simulink model "halfmodel_improved"  (R2018b)
settings: Solver=VariableStepAuto  StartTime=0.0  StopTime=10  RelTol=1e-3
values from neighbouring files (symbols this model uses):
  a = 1.25    [initModel.m]
  b = 1.4    [initModel.m]
  bodySettle = frontBodySettle-((frontBodySettle-rearBodySettle)*(a/(a+b)))    (= -0.141993301633)    [initModel.m]
  csCompress = 600    [initModel.m]
  csExtend = 1200    [initModel.m]
  frontHoldForce = mb*g*b/(a+b)    (= 2591.32075472)    [initModel.m]
  frontWheelSettle = -(frontHoldForce+(m2*g))/kT    (= -0.0199108625337)    [initModel.m]
  g = 9.81    [initModel.m]
  I = 600    [initModel.m]
  ks = 2e4    (= 20000)    [initModel.m]
  ksHard = 20*ks    (= 400000)    [initModel.m]
  kT = 14e4    (= 140000)    [initModel.m]
  kTHard = 1e10    (= 10000000000)    [initModel.m]
  m2 = 20    [initModel.m]
  mb = 500    [initModel.m]
  pitchSettle = asin((frontBodySettle-rearBodySettle)/(a+b))    [initModel.m]
  rearHoldForce = mb*g*a/(a+b)    (= 2313.67924528)    [initModel.m]
  rearWheelSettle = -(rearHoldForce+(m2*g))/kT    (= -0.0179277088949)    [initModel.m]
  stepValue = -0.2    [initModel.m]
  tyreLimit = 0.15    [initModel.m]
  v_speed = 10    [initModel.m]
  x0 = 0.2    [initModel.m]
undefined symbols (not defined in the file or in its folder): initModel
libraries: simulink x1, dspsrcs4 x1
settings Model: SnapshotBufferSize=100  Creator=Jamie  LastModifiedBy=Jamie

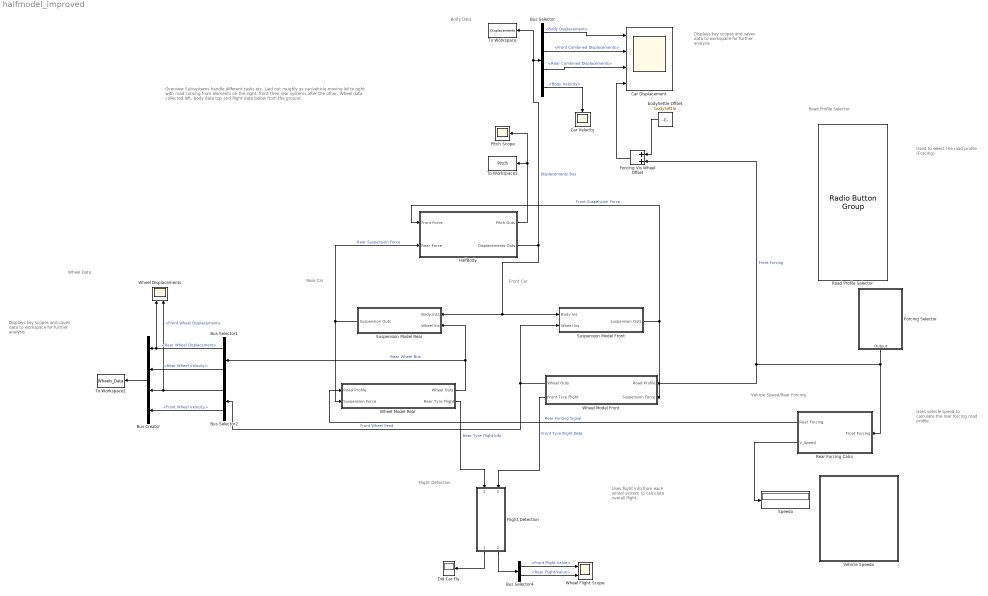
== system halfmodel_improved ==
  note: Used to select the road profile (Forcing)
  note: Vehicle Speed/Rear Forcing
  note: Flight Detection
  note: Road Profile Selector
  note: Wheel Data
  note: Front Car
  note: Rear Car
  note: Body Data
  note: Uses vehicle speed to calculate the rear forcing road profile
  note: Uses flight info from each wheel system to calculate overall flight.
  note: Displays key scopes and saves data to workspace for further analysis
  note: Displays key scopes and saves data to workspace for further analysis
  note: Overview
      | Subsystems handle different tasks etc. Laid out roughly as car/vehicle moving lef to right with road coming from elements on the right, front then rear systems after the other. Wheel data collected left, body data top and flight data below from the ground.
  Bus Creator : BusCreator  Inputs=4
  Bus Selector : BusSelector  OutputSignals=Body Displacement,Front Combined Displacements,Rear Combined Displacements,Body Velocity
  Bus Selector1 : BusSelector  OutputSignals=Rear Wheel Displacement,Rear Wheel Velocity
  Bus Selector2 : BusSelector  OutputSignals=Front Wheel Displacement,Front Wheel Velocity
  Bus Selector4 : BusSelector  OutputSignals=Front Flight Value,Rear Flight Value
  Car Displacement : Scope  NumInputPorts=4
  Car Velocity : Scope
  Did Car Fly : Display
  Flight Detection : Subsystem
  Forcing Selector : Subsystem
  Forcing Vis Wheel Offset : Sum
  HalfBody : Subsystem
  Pitch Scope : Scope
  Rear Forcing Calcs : Subsystem
  Road Profile Selector : RadioButtonGroup  LoadFcn=initModel;  WebBlockId=387  SelectedLabel=Random  ButtonGroupName=Road Input
      settings: Values={{'Step', 'Sin', 'Zero', 'Pulses', 'Humpback', 'Random'}, [1 2 3 4 5 6]}
  Speedo : Display
  Suspension Model Front : Subsystem
  Suspension Model Rear : Subsystem
  To Workspace : ToWorkspace  VariableName=Displacements  SaveFormat=Timeseries  SampleTime=-1
  To Workspace1 : ToWorkspace  VariableName=Wheels_Data  SaveFormat=Timeseries  SampleTime=-1
  To Workspace3 : ToWorkspace  VariableName=Pitch  SaveFormat=Timeseries  SampleTime=-1
  Vehicle Speedo : Subsystem  Description=Replaced Block  mask(Replaced Block){}
      mask help: This block has been replaced with an empty subsystem because it used functionality that is unavailable in Simulink R2017b.
      mask Display: fprintf('Unavailable in 2017b. \nSee report for info\nand screenshot')
  Wheel Displacements : Scope  NumInputPorts=2
  Wheel Flight Scope : Scope  NumInputPorts=2
  Wheel Model Front : Subsystem
  Wheel Model Rear : Subsystem
  bodySettle Offset : Constant  Value=bodySettle
  wires:
  HalfBody/2(Displacements Outs) -> To Workspace/1, Bus Selector/1, Suspension Model Front/1(Body Ins), Suspension Model Rear/1(Body Ins1)  "Displacements Bus"
  Suspension Model Rear/1(Suspension Outs) -> HalfBody/2(Rear Force), Wheel Model Rear/2(Suspension Force)  "Rear Suspension Force"
  Wheel Model Rear/1(Wheel Outs) -> Suspension Model Rear/2(Wheel Ins), Bus Selector1/1  "Rear Wheel Bus"
  Wheel Model Front/1(Wheel Outs) -> Bus Selector2/1, Suspension Model Front/2(Wheel Ins)  "Front Wheel Feed"
  Suspension Model Front/1(Suspension Outs) -> Wheel Model Front/2(Suspension Force), HalfBody/1(Front Force)  "Front Suspension Force"
  Forcing Selector/1(Output) -> Rear Forcing Calcs/1(Front Forcing), Forcing Vis Wheel Offset/2, Wheel Model Front/1(Road Profile)  "Front Forcing"
  Rear Forcing Calcs/1(Rear Forcing) -> Wheel Model Rear/1(Road Profile)  "Rear Forcing Signal"
  Bus Selector/4 -> Car Velocity/1  "<Body Velocity>"
  Bus Selector/1 -> Car Displacement/1  "<Body Displacement>"
  HalfBody/1(Pitch Outs) -> Pitch Scope/1, To Workspace3/1
  Bus Selector1/1 -> Wheel Displacements/1, Bus Creator/1  "<Rear Wheel Displacement>"
  Bus Selector1/2 -> Bus Creator/2  "<Rear Wheel Velocity>"
  Bus Creator/1 -> To Workspace1/1
  Bus Selector2/1 -> Wheel Displacements/2, Bus Creator/3  "<Front Wheel Displacement>"
  Bus Selector2/2 -> Bus Creator/4  "<Front Wheel Velocity>"
  Forcing Vis Wheel Offset/1 -> Car Displacement/4
  bodySettle Offset/1 -> Forcing Vis Wheel Offset/1
  Wheel Model Front/2(Front Tyre Flight) -> Flight Detection/2(Wheel 2 Data)  "Front Tyre Flight Data"
  Wheel Model Rear/2(Rear Tyre Flight) -> Flight Detection/1(Wheel 1 Data)  "Rear Tyre Flight Info"
  Flight Detection/1(Car Flight) -> Did Car Fly/1
  Flight Detection/2(Wheel Flights) -> Bus Selector4/1
  Bus Selector4/1 -> Wheel Flight Scope/1  "<Front Flight Value>"
  Bus Selector4/2 -> Wheel Flight Scope/2  "<Rear Flight Value>"
  Rear Forcing Calcs/2(V_Speed) -> Speedo/1
  Bus Selector/2 -> Car Displacement/2  "<Front Combined Displacements>"
  Bus Selector/3 -> Car Displacement/3  "<Rear Combined Displacements>"

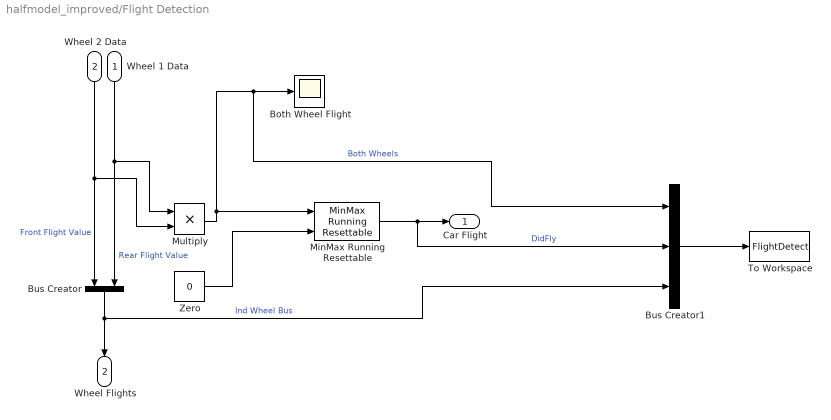
== system halfmodel_improved/Flight Detection ==
  Wheel 1 Data : Inport
  Wheel 2 Data : Inport  Port=2
  Both Wheel Flight : Scope
  Bus Creator : BusCreator  Inputs=2
  Bus Creator1 : BusCreator  Inputs=3
  MinMax Running Resettable : simulink/Math Operations/MinMax Running Resettable  Function=max  vinit=0
  Multiply : Product
  To Workspace : ToWorkspace  VariableName=FlightDetect  SaveFormat=Timeseries  SampleTime=-1
  Zero : Constant  Value=0  OutDataTypeStr=Inherit: Inherit via back propagation
  Car Flight : Outport
  Wheel Flights : Outport  Port=2
  wires:
  Wheel 1 Data/1 -> Multiply/1, Bus Creator/2  "Rear Flight Value"
  Wheel 2 Data/1 -> Multiply/2, Bus Creator/1  "Front Flight Value"
  MinMax Running Resettable/1 -> Bus Creator1/2, Car Flight/1  "DidFly"
  Multiply/1 -> Bus Creator1/1, Both Wheel Flight/1, MinMax Running Resettable/1  "Both Wheels"
  Zero/1 -> MinMax Running Resettable/2
  Bus Creator/1 -> Bus Creator1/3, Wheel Flights/1  "Ind Wheel Bus"
  Bus Creator1/1 -> To Workspace/1

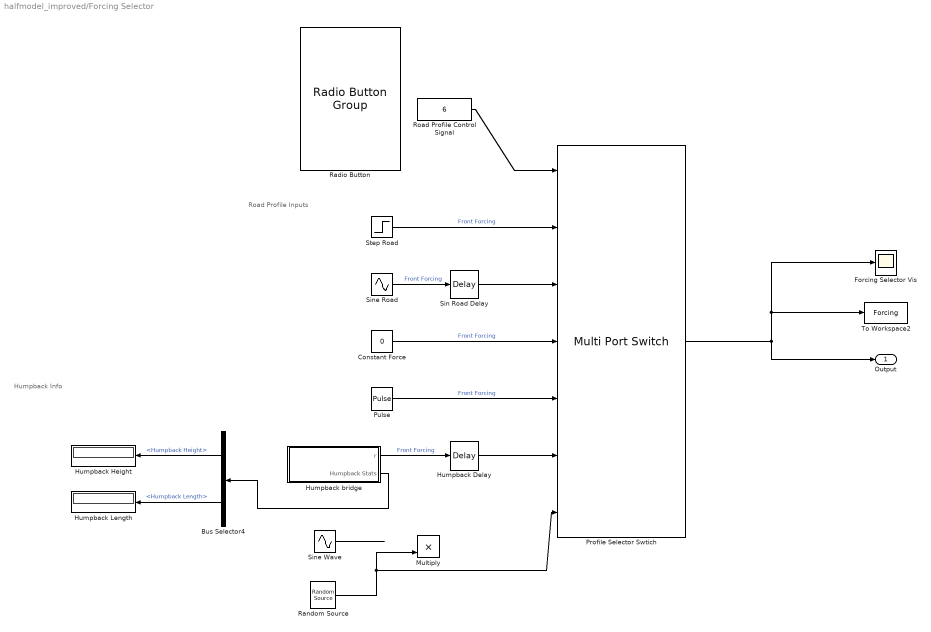
== system halfmodel_improved/Forcing Selector ==
  note: Humpback Info
  note: Road Profile Inputs
  Bus Selector4 : BusSelector  OutputSignals=Humpback Height,Humpback Length
  Constant Force : Constant  Value=0
  Forcing Selector Vis : Scope
  Humpback Delay : TransportDelay  BufferSize=4096
  Humpback bridge : Subsystem  mask{h=2, L=20, v=v_speed, startTime=0}
      mask prompts: h "humpback height (m)"; L "humpback length (m)"; v "vehicle speed (m/s)"; startTime "Humpback Start Time Multiplier"
  Humpback Height : Display
  Humpback Length : Display
  Multiply : Product
  Profile Selector Swtich : MultiPortSwitch  Inputs=6
  Pulse : DiscretePulseGenerator  PulseType=Time based  Amplitude=0.15  PulseWidth=5  PhaseDelay=1
  Radio Button : RadioButtonGroup  WebBlockId=386  SelectedLabel=Random  ButtonGroupName=Road Input
      settings: Values={{'Step', 'Sin', 'Zero', 'Pulses', 'Humpback', 'Random'}, [1 2 3 4 5 6]}
  Random Source : dspsrcs4/Random Source  SrcType=Uniform  NormMethod=Ziggurat  CltLength=12  MinVal=-0.03  MaxVal=0.03  MeanVal=0  VarVal=0.002  RepMode=Not repeatable  rawSeed=1  IsInherit=off  SampMode=Discrete  SampTime=1/20  SampFrame=1  DataType=Double  OutComplex=Real  OutputFrames=off
  Road Profile Control Signal : Constant  Value=6
  "Sin Road Delay " : TransportDelay
  Sine Road : Sin  Amplitude=0.01  Frequency=2*pi*v_speed  SampleTime=0
  Sine Wave : Sin  Frequency=2  SampleTime=0
  Step Road : Step  Time=5  After=stepValue  SampleTime=0
  To Workspace2 : ToWorkspace  VariableName=Forcing  SaveFormat=Timeseries  SampleTime=-1
  Output : Outport
  wires:
  Bus Selector4/2 -> Humpback Length/1  "<Humpback Length>"
  Bus Selector4/1 -> Humpback Height/1  "<Humpback Height>"
  Humpback bridge/2(Humpback Stats) -> Bus Selector4/1
  Step Road/1 -> Profile Selector Swtich/2  "Front Forcing"
  Sine Road/1 -> "Sin Road Delay "/1  "Front Forcing"
  Constant Force/1 -> Profile Selector Swtich/4  "Front Forcing"
  Pulse/1 -> Profile Selector Swtich/5  "Front Forcing"
  Humpback bridge/1(r) -> Humpback Delay/1  "Front Forcing"
  Road Profile Control Signal/1 -> Profile Selector Swtich/1
  Profile Selector Swtich/1 -> To Workspace2/1, Forcing Selector Vis/1, Output/1
  Humpback Delay/1 -> Profile Selector Swtich/6
  "Sin Road Delay "/1 -> Profile Selector Swtich/3
  Sine Wave/1 -> ?
  Random Source/1 -> Multiply/2, Profile Selector Swtich/7

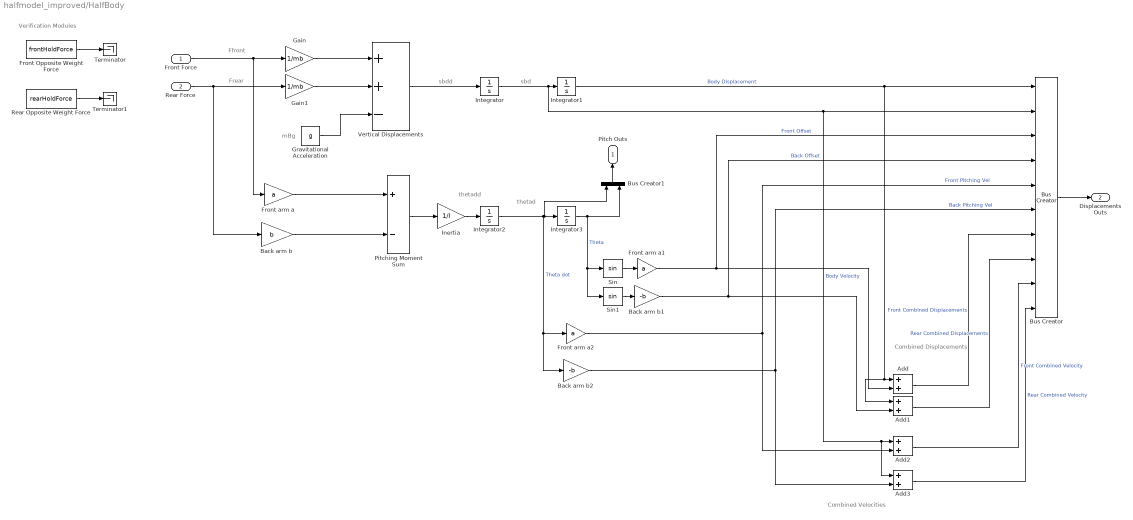
== system halfmodel_improved/HalfBody ==
  note: Combined Velocities
  note: Verification Modules
  note: thetadd
  note: Ffront
  note: Frear
  note: mBg
  note: sbdd
  note: sbd
  note: thetad
  note: Combined
      | Displacements
  Front Force : Inport
  Rear Force : Inport  Port=2
  Add{,1..3} (4 alike) : Sum
  Back arm b : Gain  Gain=b
  Back arm b1 : Gain  Gain=-b
  Back arm b2 : Gain  Gain=-b
  Bus Creator : BusCreator  Inputs=10
  Bus Creator1 : BusCreator  Inputs=2
  Front Opposite Weight Force : Constant  Value=frontHoldForce
  Front arm a : Gain  Gain=a
  Front arm a1 : Gain  Gain=a
  Front arm a2 : Gain  Gain=a
  Gain : Gain  Gain=1/mb
  Gain1 : Gain  Gain=1/mb
  Gravitational Acceleration : Constant  Value=g  mask{g=g}
      mask prompts: g "Gravitational Acceleration"
  Inertia : Gain  Gain=1/I
  Integrator : Integrator
  Integrator1 : Integrator  InitialCondition=bodySettle
  Integrator2 : Integrator
  Integrator3 : Integrator  InitialCondition=pitchSettle
  Pitching Moment Sum : Sum  Inputs=+-
  Rear Opposite Weight Force : Constant  Value=rearHoldForce
  Sin : Trigonometry
  Sin1 : Trigonometry
  Terminator : Terminator
  Terminator1 : Terminator
  Vertical Displacements : Sum  Inputs=++-
  Pitch Outs : Outport
  Displacements Outs : Outport  Port=2
  wires:
  Gravitational Acceleration/1 -> Vertical Displacements/3
  Gain/1 -> Vertical Displacements/1
  Gain1/1 -> Vertical Displacements/2
  Integrator1/1 -> Bus Creator/1, Add1/1, Add/1  "Body Displacement"
  Vertical Displacements/1 -> Integrator/1
  Integrator/1 -> Add2/1, Add3/1, Bus Creator/2, Integrator1/1  "Body Velocity"
  Back arm b/1 -> Pitching Moment Sum/2
  Front arm a/1 -> Pitching Moment Sum/1
  Pitching Moment Sum/1 -> Inertia/1
  Integrator2/1 -> Back arm b2/1, Front arm a2/1, Integrator3/1, Bus Creator1/1  "Theta dot"
  Inertia/1 -> Integrator2/1
  Bus Creator1/1 -> Pitch Outs/1
  Integrator3/1 -> Bus Creator1/2, Sin1/1, Sin/1  "Theta"
  Front arm a1/1 -> Add/2, Bus Creator/3  "Front Offset"
  Back arm b1/1 -> Add1/2, Bus Creator/4  "Back Offset"
  Bus Creator/1 -> Displacements Outs/1
  Front arm a2/1 -> Bus Creator/5, Add2/2  "Front Pitching Vel"
  Back arm b2/1 -> Bus Creator/6, Add3/2  "Back Pitching Vel"
  Sin/1 -> Front arm a1/1
  Sin1/1 -> Back arm b1/1
  Rear Force/1 -> Back arm b/1, Gain1/1
  Front Force/1 -> Gain/1, Front arm a/1
  Front Opposite Weight Force/1 -> Terminator/1
  Rear Opposite Weight Force/1 -> Terminator1/1
  Add/1 -> Bus Creator/7  "Front Combined Displacements"
  Add1/1 -> Bus Creator/8  "Rear Combined Displacements"
  Add2/1 -> Bus Creator/9  "Front Combined Velocity"
  Add3/1 -> Bus Creator/10  "Rear Combined Velocity"

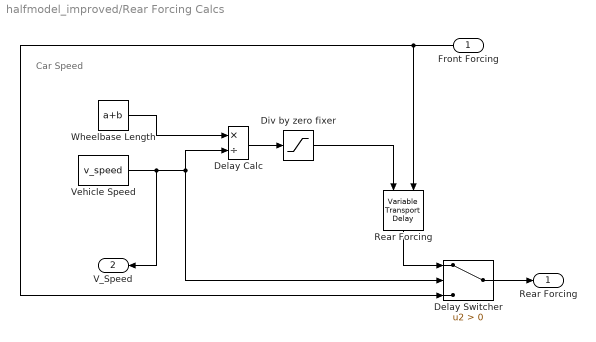
== system halfmodel_improved/Rear Forcing Calcs ==
  note: Car Speed
  Front Forcing : Inport
  Delay Calc : Product  Inputs=*/
  Delay Switcher : Switch  Criteria=u2 > Threshold
  Div by zero fixer : Saturate  UpperLimit=60  LowerLimit=0
  "Rear Forcing " : VariableTransportDelay  VariableDelayType=Variable transport delay  MaximumDelay=60  MaximumPoints=8192
  Vehicle Speed : Constant  Value=v_speed
  Wheelbase Length : Constant  Value=a+b
  Rear Forcing : Outport
  V_Speed : Outport  Port=2
  wires:
  Vehicle Speed/1 -> V_Speed/1, Delay Switcher/2, Delay Calc/2
  Delay Calc/1 -> Div by zero fixer/1
  Front Forcing/1 -> "Rear Forcing "/1, Delay Switcher/3
  Delay Switcher/1 -> Rear Forcing/1
  Wheelbase Length/1 -> Delay Calc/1
  "Rear Forcing "/1 -> Delay Switcher/1
  Div by zero fixer/1 -> "Rear Forcing "/2

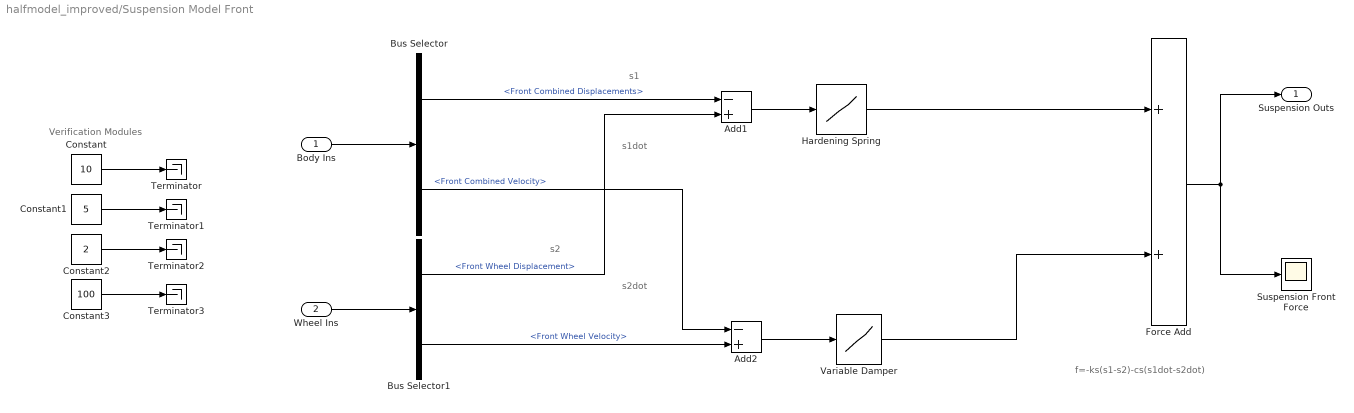
== system halfmodel_improved/Suspension Model Front ==
  note: Verification Modules
  note: s2dot
  note: s2
  note: f=-ks(s1-s2)-cs(s1dot-s2dot)
  note: s1dot
  note: s1
  Body Ins : Inport
  Wheel Ins : Inport  Port=2
  Add1 : Sum  Inputs=-+
  Add2 : Sum  Inputs=-+
  Bus Selector : BusSelector  OutputSignals=Front Combined Displacements,Front Combined Velocity
  Bus Selector1 : BusSelector  OutputSignals=Front Wheel Displacement,Front Wheel Velocity
  Constant : Constant  Value=10
  Constant1 : Constant  Value=5
  Constant2 : Constant  Value=2
  Constant3 : Constant  Value=100
  "Force Add " : Sum
  Hardening Spring : Lookup_n-D  NumberOfTableDimensions=1  BreakpointsForDimension1=[-2*x0,-1.5*x0,-x0,x0,1.5*x0,2*x0]  Table=[-1e10,-(ks+(ksHard/2))*x0,-ks*x0,ks*x0,(ks+(ksHard/2))*x0,1e10]  InternalRulePriority=Speed  RndMeth=Simplest  InputSameDT=on
  Suspension Front Force : Scope
  Terminator{,1..3} (4 alike) : Terminator
  Variable Damper : Lookup_n-D  NumberOfTableDimensions=1  BreakpointsForDimension1=[-1,0,1]  Table=[-csExtend,0,csCompress]  InternalRulePriority=Speed  RndMeth=Simplest  InputSameDT=on
  Suspension Outs : Outport
  wires:
  Body Ins/1 -> Bus Selector/1
  Wheel Ins/1 -> Bus Selector1/1
  Bus Selector1/2 -> Add2/2  "<Front Wheel Velocity>"
  Bus Selector1/1 -> Add1/2  "<Front Wheel Displacement>"
  "Force Add "/1 -> Suspension Front Force/1, Suspension Outs/1
  Bus Selector/1 -> Add1/1  "<Front Combined Displacements>"
  Bus Selector/2 -> Add2/1  "<Front Combined Velocity>"
  Constant/1 -> Terminator/1
  Constant1/1 -> Terminator1/1
  Constant2/1 -> Terminator2/1
  Constant3/1 -> Terminator3/1
  Hardening Spring/1 -> "Force Add "/1
  Add2/1 -> Variable Damper/1
  Variable Damper/1 -> "Force Add "/2
  Add1/1 -> Hardening Spring/1

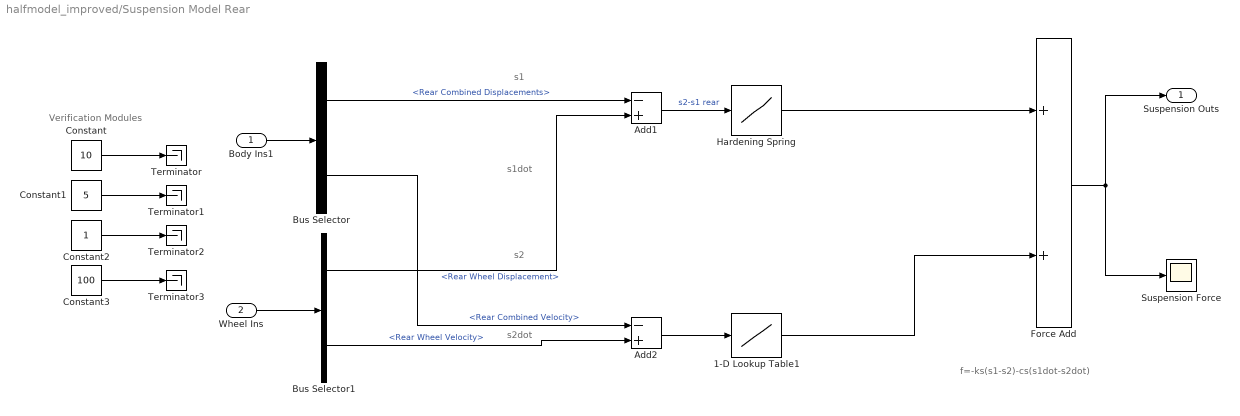
== system halfmodel_improved/Suspension Model Rear ==
  note: Verification Modules
  note: s2dot
  note: s2
  note: f=-ks(s1-s2)-cs(s1dot-s2dot)
  note: s1dot
  note: s1
  Body Ins1 : Inport
  Wheel Ins : Inport  Port=2
  1-D Lookup Table1 : Lookup_n-D  NumberOfTableDimensions=1  BreakpointsForDimension1=[-1,0,1]  Table=[-csExtend,0,csCompress]  InternalRulePriority=Speed  RndMeth=Simplest  InputSameDT=on
  Add1 : Sum  Inputs=-+
  Add2 : Sum  Inputs=-+
  Bus Selector : BusSelector  OutputSignals=Rear Combined Displacements,Rear Combined Velocity
  Bus Selector1 : BusSelector  OutputSignals=Rear Wheel Displacement,Rear Wheel Velocity
  Constant : Constant  Value=10
  Constant1 : Constant  Value=5
  Constant2 : Constant
  Constant3 : Constant  Value=100
  "Force Add " : Sum
  Hardening Spring : Lookup_n-D  NumberOfTableDimensions=1  BreakpointsForDimension1=[-2*x0,-1.5*x0,-x0,x0,1.5*x0,2*x0]  Table=[-1e10,-(ks+(ksHard/2))*x0,-ks*x0,ks*x0,(ks+(ksHard/2))*x0,1e10]  InternalRulePriority=Speed  RndMeth=Simplest  InputSameDT=on
  Suspension Force : Scope
  Terminator{,1..3} (4 alike) : Terminator
  Suspension Outs : Outport
  wires:
  Bus Selector1/2 -> Add2/2  "<Rear Wheel Velocity>"
  Bus Selector1/1 -> Add1/2  "<Rear Wheel Displacement>"
  "Force Add "/1 -> Suspension Force/1, Suspension Outs/1
  Body Ins1/1 -> Bus Selector/1
  Bus Selector/1 -> Add1/1  "<Rear Combined Displacements>"
  Wheel Ins/1 -> Bus Selector1/1
  Constant3/1 -> Terminator3/1
  Constant1/1 -> Terminator1/1
  Constant2/1 -> Terminator2/1
  Constant/1 -> Terminator/1
  1-D Lookup Table1/1 -> "Force Add "/2
  Hardening Spring/1 -> "Force Add "/1
  Add2/1 -> 1-D Lookup Table1/1
  Add1/1 -> Hardening Spring/1  "s2-s1 rear"
  Bus Selector/2 -> Add2/1  "<Rear Combined Velocity>"

== system halfmodel_improved/Vehicle Speedo ==

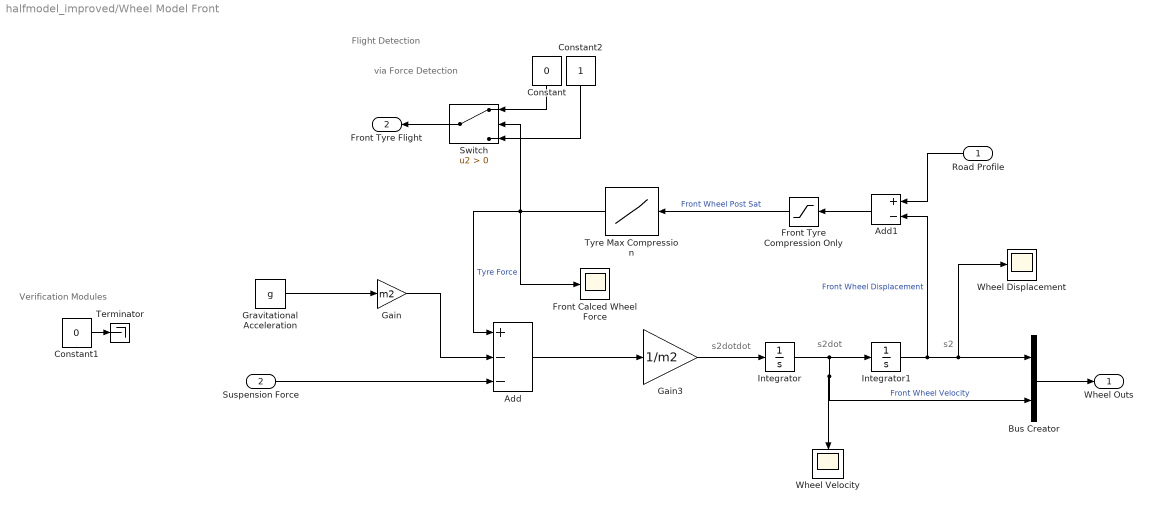
== system halfmodel_improved/Wheel Model Front ==
  note: Verification Modules
  note: Flight Detection
  note: s2
  note: s2dot
  note: s2dotdot
  note: via Force Detection
  Road Profile : Inport
  Suspension Force : Inport  Port=2
  Add : Sum  Inputs=+--
  Add1 : Sum  Inputs=+-
  Bus Creator : BusCreator  Inputs=2
  Constant : Constant  Value=0
  Constant1 : Constant  Value=0
  Constant2 : Constant
  Front Calced Wheel Force : Scope
  Front Tyre Compression Only : Saturate  UpperLimit=inf  LowerLimit=0
  Gain : Gain  Gain=m2
  Gain3 : Gain  Gain=1/m2
  Gravitational Acceleration : Constant  Value=g  mask{g=g}
      mask prompts: g "Gravitatioanl Acceleration"
  Integrator : Integrator
  Integrator1 : Integrator  InitialCondition=frontWheelSettle
  Switch : Switch  Criteria=u2 > Threshold
  Terminator : Terminator
  Tyre Max Compression : Lookup_n-D  NumberOfTableDimensions=1  BreakpointsForDimension1=[0, tyreLimit, 2*tyreLimit]  Table=[0,tyreLimit*kT,2*tyreLimit*kTHard]  InternalRulePriority=Speed  RndMeth=Simplest  InputSameDT=on
  Wheel Displacement : Scope
  Wheel Velocity : Scope
  Wheel Outs : Outport
  Front Tyre Flight : Outport  Port=2
  wires:
  Road Profile/1 -> Add1/1
  Gravitational Acceleration/1 -> Gain/1
  Gain3/1 -> Integrator/1
  Integrator/1 -> Bus Creator/2, Wheel Velocity/1, Integrator1/1  "Front Wheel Velocity"
  Integrator1/1 -> Add1/2, Wheel Displacement/1, Bus Creator/1  "Front Wheel Displacement"
  Bus Creator/1 -> Wheel Outs/1
  Add/1 -> Gain3/1
  Gain/1 -> Add/2
  Suspension Force/1 -> Add/3
  Tyre Max Compression/1 -> Switch/2, Front Calced Wheel Force/1, Add/1  "Tyre Force"
  Add1/1 -> Front Tyre Compression Only/1
  Front Tyre Compression Only/1 -> Tyre Max Compression/1  "Front Wheel Post Sat"
  Constant1/1 -> Terminator/1
  Constant/1 -> Switch/1
  Constant2/1 -> Switch/3
  Switch/1 -> Front Tyre Flight/1

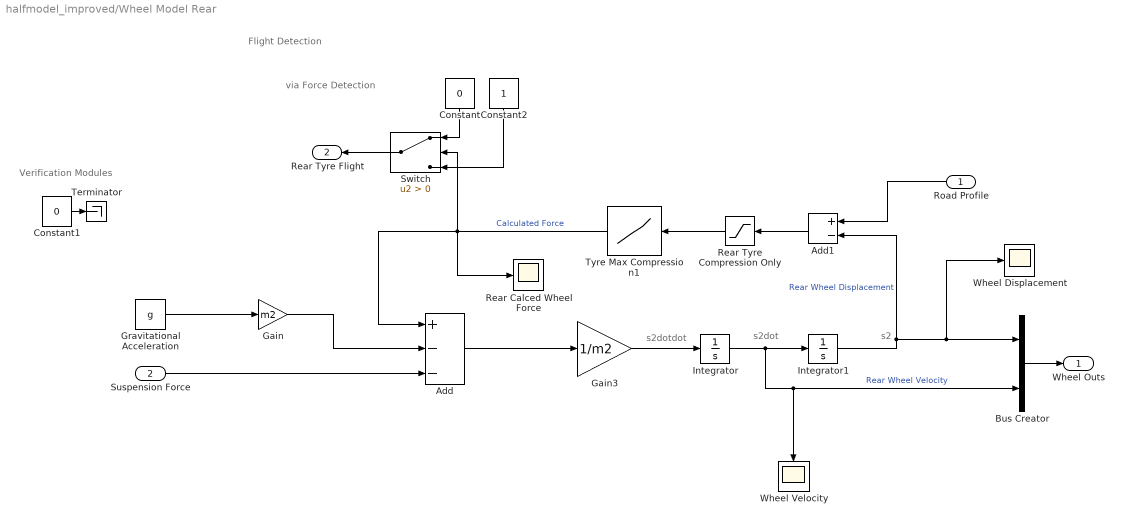
== system halfmodel_improved/Wheel Model Rear ==
  note: via Force Detection
  note: Flight Detection
  note: Verification Modules
  note: s2
  note: s2dot
  note: s2dotdot
  Road Profile : Inport
  Suspension Force : Inport  Port=2
  Add : Sum  Inputs=+--
  Add1 : Sum  Inputs=+-
  Bus Creator : BusCreator  Inputs=2
  Constant : Constant  Value=0
  Constant1 : Constant  Value=0
  Constant2 : Constant
  Gain : Gain  Gain=m2
  Gain3 : Gain  Gain=1/m2
  Gravitational Acceleration : Constant  Value=g  mask{g=g}
      mask prompts: g "Gravitatioanl Acceleration"
  Integrator : Integrator
  Integrator1 : Integrator  InitialCondition=rearWheelSettle
  Rear Calced Wheel Force : Scope
  Rear Tyre Compression Only : Saturate  UpperLimit=inf  LowerLimit=0
  Switch : Switch  Criteria=u2 > Threshold
  Terminator : Terminator
  Tyre Max Compression1 : Lookup_n-D  NumberOfTableDimensions=1  BreakpointsForDimension1=[0, tyreLimit, 2*tyreLimit]  Table=[0,tyreLimit*kT,2*tyreLimit*kTHard]  InternalRulePriority=Speed  RndMeth=Simplest  InputSameDT=on
  Wheel Displacement : Scope
  Wheel Velocity : Scope
  Wheel Outs : Outport
  Rear Tyre Flight : Outport  Port=2
  wires:
  Gravitational Acceleration/1 -> Gain/1
  Gain3/1 -> Integrator/1
  Integrator/1 -> Wheel Velocity/1, Bus Creator/2, Integrator1/1  "Rear Wheel Velocity"
  Bus Creator/1 -> Wheel Outs/1
  Add/1 -> Gain3/1
  Gain/1 -> Add/2
  Suspension Force/1 -> Add/3
  Road Profile/1 -> Add1/1
  Integrator1/1 -> Add1/2, Wheel Displacement/1, Bus Creator/1  "Rear Wheel Displacement"
  Rear Tyre Compression Only/1 -> Tyre Max Compression1/1
  Add1/1 -> Rear Tyre Compression Only/1
  Constant1/1 -> Terminator/1
  Switch/1 -> Rear Tyre Flight/1
  Constant/1 -> Switch/1
  Tyre Max Compression1/1 -> Rear Calced Wheel Force/1, Switch/2, Add/1  "Calculated Force"
  Constant2/1 -> Switch/3

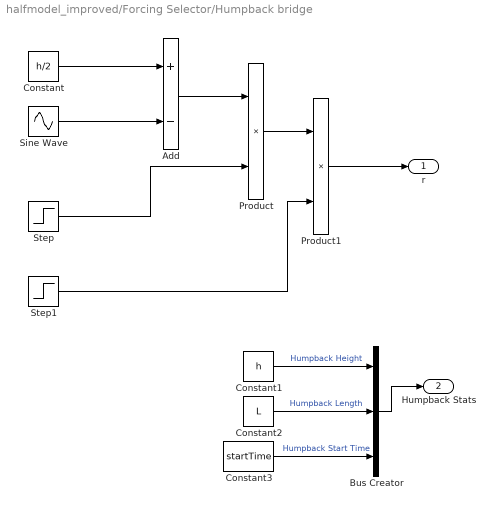
== system halfmodel_improved/Forcing Selector/Humpback bridge ==
  Add : Sum  Inputs=+-
  Bus Creator : BusCreator  Inputs=3
  Constant : Constant  Value=h/2
  Constant1 : Constant  Value=h
  Constant2 : Constant  Value=L
  Constant3 : Constant  Value=startTime
  Product : Product
  Product1 : Product
  Sine Wave : Sin  Amplitude=h/2  Frequency=2*pi*v/L  Phase=pi/2  SampleTime=0
  Step : Step  Time=startTime*L/max(v,0.01)  SampleTime=0
  Step1 : Step  Time=(startTime+1)*L/max(v,0.01)  Before=1  After=0  SampleTime=0
  r : Outport
  Humpback Stats : Outport  Port=2
  wires:
  Constant/1 -> Add/1
  Sine Wave/1 -> Add/2
  Add/1 -> Product/1
  Step/1 -> Product/2
  Product/1 -> Product1/1
  Step1/1 -> Product1/2
  Product1/1 -> r/1
  Constant1/1 -> Bus Creator/1  "Humpback Height"
  Constant2/1 -> Bus Creator/2  "Humpback Length"
  Bus Creator/1 -> Humpback Stats/1
  Constant3/1 -> Bus Creator/3  "Humpback Start Time"
